simulink model "Exp1_pendulum"  (R2023b)
settings: Solver=ode3  StartTime=0.0  StopTime=10.0  FixedStep=0.001  RelTol=1e-3
values from neighbouring files (symbols this model uses):
  d = m * g * l * (cos(phi_2) - cos(phi_1)) / Integral    [Exp1_estimation_d.m]    (also in Exp1_parameters_steel_math.m = 0.00266991944412; Exp1_parameters_steel_phys.m = 0.00274110004552; Exp1_parameters_styrofoam_math.m = 0.000186312591304; Exp1_parameters_styrofoam_phys.m = 0.00166165647764)
  g = 9.81    [Exp1_parameters_steel_math.m]    (also in Exp1_parameters_steel_phys.m; Exp1_parameters_styrofoam_math.m; Exp1_parameters_styrofoam_phys.m)
  J = m*l^2    (= 0.4942189)    [Exp1_parameters_steel_math.m]    (also in Exp1_parameters_steel_phys.m = 0.503352452; Exp1_parameters_styrofoam_math.m = 0.0016639175; Exp1_parameters_styrofoam_phys.m = 0.0101157325)
  l = l_R - s + r_B    (= 0.595)    [Exp1_parameters_steel_math.m]    (also in Exp1_parameters_steel_phys.m = 0.455123285478; Exp1_parameters_styrofoam_math.m; Exp1_parameters_styrofoam_phys.m = 0.051701907131)
  m = m_B    (= 1.396)    [Exp1_parameters_steel_math.m]    (also in Exp1_parameters_steel_phys.m = 1.8737; Exp1_parameters_styrofoam_math.m = 0.0047; Exp1_parameters_styrofoam_phys.m = 0.4824)
settings Model: Creator=shaunclarenceraj  LastModifiedBy=dain

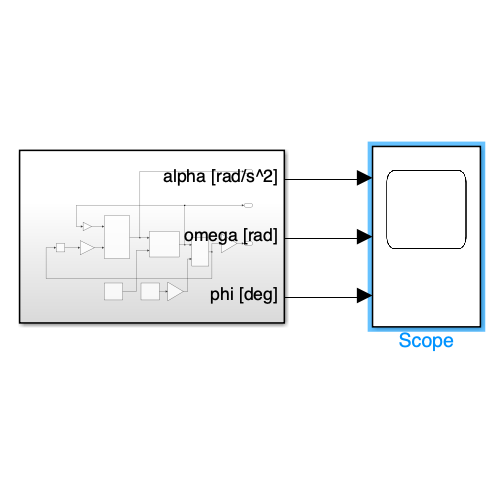
[thumbnail: Simulink's stored preview of the top-level diagram]
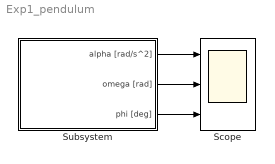
== system Exp1_pendulum ==
  Scope : Scope  NumInputPorts=3
  Subsystem : Subsystem
  wires:
  Subsystem/1(alpha [rad/s^2]) -> Scope/1
  Subsystem/2(omega [rad]) -> Scope/2
  Subsystem/3(phi [deg]) -> Scope/3

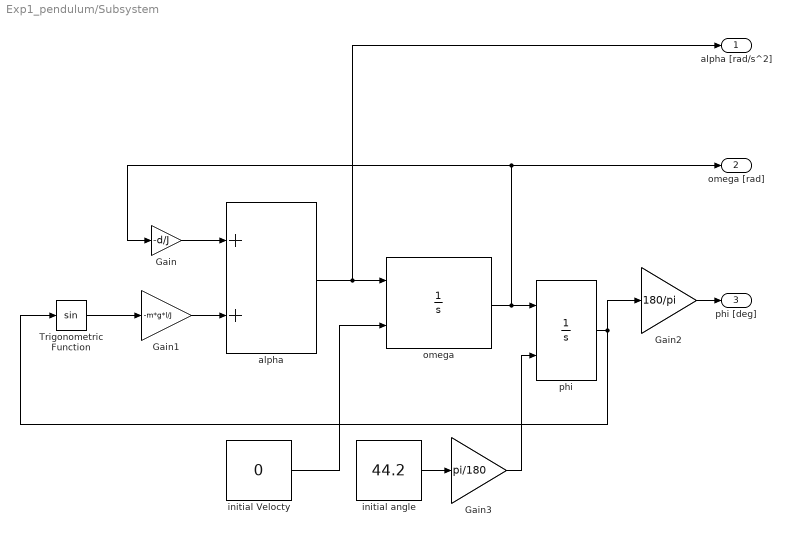
== system Exp1_pendulum/Subsystem ==
  Gain : Gain  Gain=-d/J
  Gain1 : Gain  Gain=-m*g*l/J
  Gain2 : Gain  Gain=180/pi
  Gain3 : Gain  Gain=pi/180
  Trigonometric Function : Trigonometry
  alpha : Sum
  "initial Velocty " : Constant  Value=0
  initial angle : Constant  Value=44.2
  omega : Integrator  InitialConditionSource=external
  phi : Integrator  InitialConditionSource=external
  alpha [rad/s^2] : Outport
  omega [rad] : Outport  Port=2
  phi [deg] : Outport  Port=3
  wires:
  alpha/1 -> omega/1, alpha [rad/s^2]/1
  "initial Velocty "/1 -> omega/2
  Gain/1 -> alpha/1
  Gain1/1 -> alpha/2
  phi/1 -> Gain2/1, Trigonometric Function/1
  omega/1 -> omega [rad]/1, Gain/1, phi/1
  Gain2/1 -> phi [deg]/1
  Trigonometric Function/1 -> Gain1/1
  initial angle/1 -> Gain3/1
  Gain3/1 -> phi/2
